simulink model "toggle_flip_flop"  (R2018a)
settings: Solver=VariableStepAuto  StartTime=0.0  StopTime=10.0  RelTol=1e-3
libraries: simulink_extras x1
settings Model: Creator=Edoardo  LastModifiedBy=Edoardo

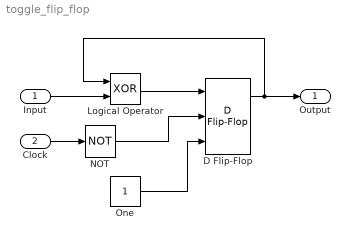
== system toggle_flip_flop ==
  Input : Inport
  Clock : Inport  Port=2  OutDataTypeStr=boolean
  D Flip-Flop : simulink_extras/Flip Flops/D Flip-Flop
      settings: SourceProductName=Simulink
  Logical Operator : Logic  Operator=XOR  AllPortsSameDT=off  OutDataTypeStr=boolean
  NOT : Logic  Operator=NOT  IconShape=distinctive  AllPortsSameDT=off  OutDataTypeStr=boolean
  One : Constant
  Output : Outport
  wires:
  Input/1 -> Logical Operator/2
  Clock/1 -> NOT/1
  D Flip-Flop/1 -> Output/1, Logical Operator/1
  Logical Operator/1 -> D Flip-Flop/1
  One/1 -> D Flip-Flop/3
  NOT/1 -> D Flip-Flop/2
